simulink model "lab4"  (R2015a)
settings: Solver=ode45  StartTime=0.0  StopTime=1000.0  RelTol=1e-3
values from neighbouring files (symbols this model uses):
  K = 0.08    [lab4.m]
  Ti = 200    [lab4.m]
  Tr = 1    [lab4.m]
  Ts = 16.4    [lab4.m]
settings Model: Creator=vbox  LastModifiedBy=vbox
settings DataIOCC: InspectSignalLogs=on

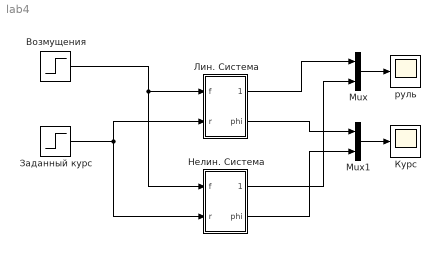
== system lab4 ==
  Mux : Mux  Inputs=2
  Mux1 : Mux  Inputs=2
  Возмущения : Step  After=2  SampleTime=0
  Заданный курс : Step  Time=0  After=90  SampleTime=0
  Курс : Scope
      settings: SaveName=phi
  Лин. Система : Subsystem
  Нелин. Система : Subsystem
  руль : Scope
      settings: TimeRange=100  YMin=-10  YMax=70  SaveName=delta
  wires:
  Mux/1 -> руль/1
  Mux1/1 -> Курс/1
  Лин. Система/1(delta) -> Mux/1
  Нелин. Система/1(delta) -> Mux/2
  Лин. Система/2(phi) -> Mux1/1
  Нелин. Система/2(phi) -> Mux1/2
  Возмущения/1 -> Лин. Система/1(f), Нелин. Система/1(f)
  Заданный курс/1 -> Лин. Система/2(r), Нелин. Система/2(r)

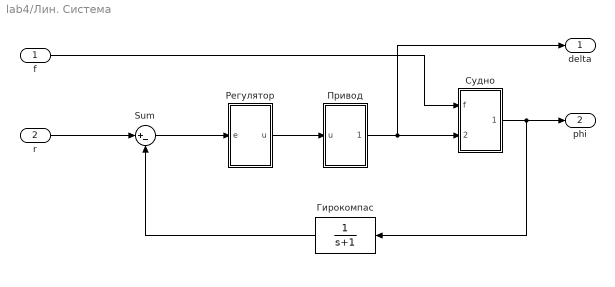
== system lab4/Лин. Система ==
  f : Inport
  r : Inport  Port=2
  Sum : Sum  Inputs=|+-
  Гирокомпас : TransferFcn  Denominator=[1 1]
  Привод : Subsystem
  Регулятор : Subsystem
  Судно : Subsystem
  delta : Outport
  phi : Outport  Port=2
  wires:
  Гирокомпас/1 -> Sum/2
  r/1 -> Sum/1
  Судно/1(phi) -> phi/1, Гирокомпас/1
  Sum/1 -> Регулятор/1(e)
  f/1 -> Судно/1(f)
  Привод/1(delta) -> delta/1, Судно/2(delta)
  Регулятор/1(u) -> Привод/1(u)

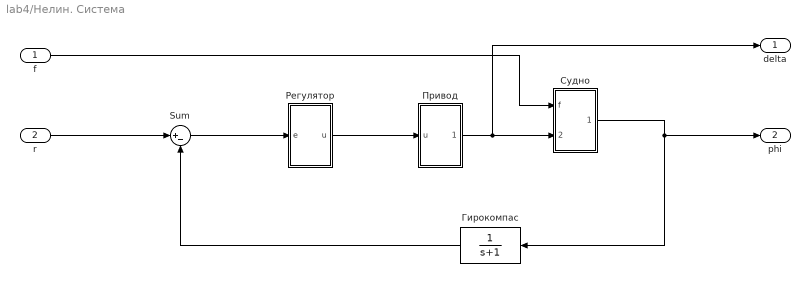
== system lab4/Нелин. Система ==
  f : Inport
  r : Inport  Port=2
  Sum : Sum  Inputs=|+-
  Гирокомпас : TransferFcn  Denominator=[1 1]
  Привод : Subsystem
  Регулятор : Subsystem
  Судно : Subsystem
  delta : Outport
  phi : Outport  Port=2
  wires:
  Гирокомпас/1 -> Sum/2
  r/1 -> Sum/1
  Судно/1(phi) -> phi/1, Гирокомпас/1
  Sum/1 -> Регулятор/1(e)
  f/1 -> Судно/1(f)
  Привод/1(delta) -> delta/1, Судно/2(delta)
  Регулятор/1(u) -> Привод/1(u)

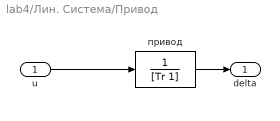
== system lab4/Лин. Система/Привод ==
  u : Inport
  привод : TransferFcn  Denominator=[Tr 1]
  delta : Outport
  wires:
  привод/1 -> delta/1
  u/1 -> привод/1

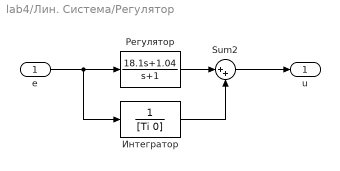
== system lab4/Лин. Система/Регулятор ==
  e : Inport
  Sum2 : Sum  Inputs=|++
  Интегратор : TransferFcn  Denominator=[Ti 0]
  Регулятор : TransferFcn  Numerator=[18.1 1.04]  Denominator=[1 1]
  u : Outport
  wires:
  e/1 -> Интегратор/1, Регулятор/1
  Sum2/1 -> u/1
  Регулятор/1 -> Sum2/1
  Интегратор/1 -> Sum2/2

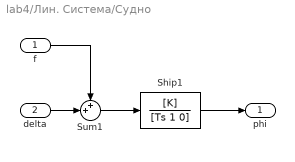
== system lab4/Лин. Система/Судно ==
  f : Inport
  delta : Inport  Port=2
  Ship1 : TransferFcn  Numerator=[K]  Denominator=[Ts 1 0]
  Sum1 : Sum  Inputs=++|
  phi : Outport
  wires:
  Sum1/1 -> Ship1/1
  Ship1/1 -> phi/1
  f/1 -> Sum1/1
  delta/1 -> Sum1/2

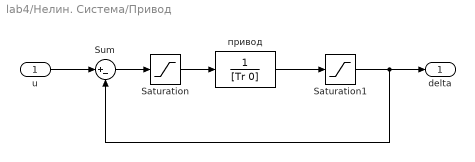
== system lab4/Нелин. Система/Привод ==
  u : Inport
  Saturation : Saturate  UpperLimit=3  LowerLimit=-3
      settings: LockScale=on
  Saturation1 : Saturate  UpperLimit=50  LowerLimit=-50
  Sum : Sum  Inputs=|+-
  привод : TransferFcn  Denominator=[Tr 0]
  delta : Outport
  wires:
  u/1 -> Sum/1
  Sum/1 -> Saturation/1
  Saturation/1 -> привод/1
  привод/1 -> Saturation1/1
  Saturation1/1 -> Sum/2, delta/1

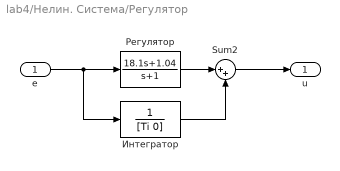
== system lab4/Нелин. Система/Регулятор ==
  e : Inport
  Sum2 : Sum  Inputs=|++
  Интегратор : TransferFcn  Denominator=[Ti 0]
  Регулятор : TransferFcn  Numerator=[18.1 1.04]  Denominator=[1 1]
  u : Outport
  wires:
  e/1 -> Интегратор/1, Регулятор/1
  Sum2/1 -> u/1
  Регулятор/1 -> Sum2/1
  Интегратор/1 -> Sum2/2

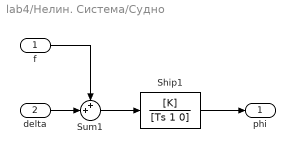
== system lab4/Нелин. Система/Судно ==
  f : Inport
  delta : Inport  Port=2
  Ship1 : TransferFcn  Numerator=[K]  Denominator=[Ts 1 0]
  Sum1 : Sum  Inputs=++|
  phi : Outport
  wires:
  Sum1/1 -> Ship1/1
  Ship1/1 -> phi/1
  f/1 -> Sum1/1
  delta/1 -> Sum1/2
